simulink model "MotorX_modelling"  (R2020a)
settings: Solver=FixedStepAuto  StartTime=0.0  StopTime=10  RelTol=1e-3  EnableMultiTasking=on
libraries: arduinolib x6, simulink x3, arduinosensorlib x1
settings Model: SILPILModeSetting=veronly  ExtModeTrigDuration=2  Creator=fcemi  LastModifiedBy=fcemi
settings OptimizationCC: EnhancedBackFolding=on  PassReuseOutputArgsAs=Individual arguments  ZeroExternalMemoryAtStartup=off  ZeroInternalMemoryAtStartup=off  MaxStackSize=64  OptimizeBlockOrder=speed  DifferentSizesBufferReuse=on  OptimizationCustomize=off  EfficientTunableParamExpr=on
settings DebuggingCC: ParameterTunabilityLossMsg=error
settings HardwareCC: ProdBitPerInt=16  ProdBitPerPointer=16  ProdBitPerSizeT=16  ProdBitPerPtrDiffT=16  ProdLargestAtomicFloat=None  ProdWordSize=8  ProdHWDeviceType=Atmel->AVR  UseEmbeddedCoderFeatures=off  UseSimulinkCoderFeatures=off
settings SFSimCC: MATLABDynamicMemAlloc=off
settings RTWCC: SystemTargetFile=ert.tlc  HardwareBoard=Arduino Uno  TLCOptions=-aInlineSetEventsForThisBaseRateFcn=TLC_FALSE -aSuppressMultiTaskScheduler=TLC_FALSE -aRateBasedStepFcn=1  TemplateMakefile=ert_default_tmf  Toolchain=Arduino AVR  BuildConfiguration=Faster Runs
settings CodeAppCC: ForceParamTrailComments=on  IgnoreCustomStorageClasses=off  OperatorAnnotations=on  SimulinkDataObjDesc=on  SFDataObjDesc=on  InsertBlockDesc=on
settings ERTTargetCC: SupportContinuousTime=on  SupportNonInlinedSFcns=on  SupportVariableSizeSignals=on  ExtModeStaticAllocSize=250

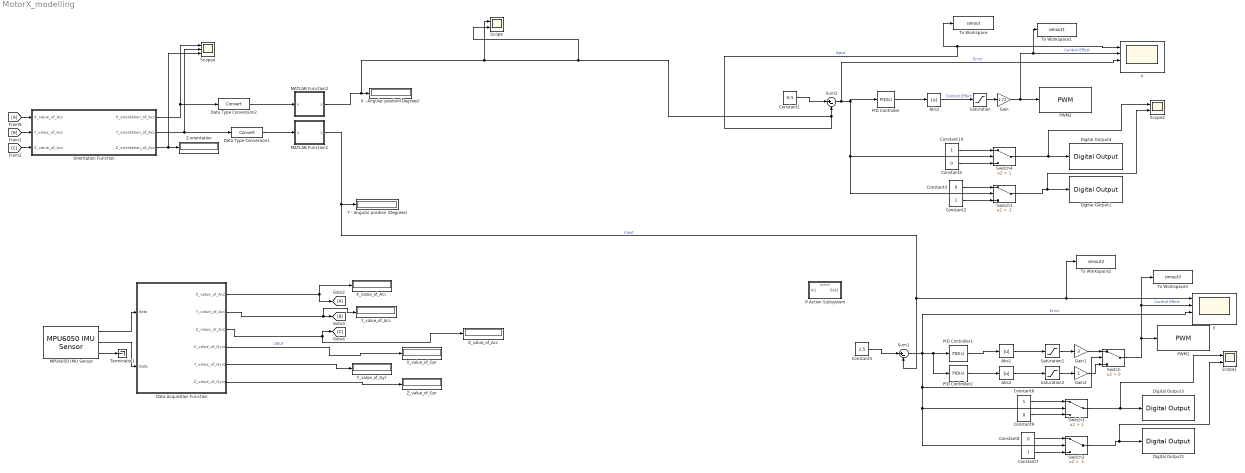
== system MotorX_modelling ==
  Abs1 : Abs
  Abs2 : Abs
  Abs3 : Abs
  Constant1 : Constant  Value=-0.5
  Constant{2,6..7,10} (4 alike) : Constant
  Constant{3..4,8..9} (4 alike) : Constant  Value=0
  Constant5 : Constant  Value=2.5
  Data Acquisition Function : MATLAB Function  TreatAsAtomicUnit=on
  Data Type Conversion1 : DataTypeConversion
  Data Type Conversion2 : DataTypeConversion
  Digital Output1 : arduinolib/Digital Output  pinNumber=8  Direction=output  blockPlatform=arduino
  Digital Output2 : arduinolib/Digital Output  pinNumber=5  Direction=output  blockPlatform=arduino
  Digital Output3 : arduinolib/Digital Output  pinNumber=4  Direction=output  blockPlatform=arduino
  Digital Output4 : arduinolib/Digital Output  pinNumber=9  Direction=output  blockPlatform=arduino
  Gain : Gain  Gain=1.72
  Gain1 : Gain  Gain=3
  Gain2 : Gain
  If Action Subsystem : Subsystem  TreatAsAtomicUnit=on
  MATLAB Function1 : MATLAB Function  TreatAsAtomicUnit=on
  MATLAB Function2 : MATLAB Function  TreatAsAtomicUnit=on
  MPU6050 IMU Sensor : arduinosensorlib/MPU6050 IMU Sensor  SlaveAddress=0x68  Accel=on  AngularRate=on  Temperature=off  Status=on  EulerAngles=off  Quat=off  AccelRange=2G  GyroRange=250 dps  DmpOdr=200 Hz  Dlpf=Accelerometer: 184Hz, Gyroscope: 188Hz  SampleTime=0.01
      settings: SourceProductBaseCode=ARDUINO
  Orientation Function : MATLAB Function  TreatAsAtomicUnit=on
  PID Controller : simulink/Continuous/PID Controller  Controller=PID  Form=Parallel  TimeDomain=Continuous-time  UseExternalTs=off  SampleTime=-1  IntegratorMethod=Forward Euler  FilterMethod=Forward Euler  ControllerParametersSource=internal  P=1  I=0  D=0.01  UseFilter=on  N=100  TunerSelectOption=Transfer Function Based (PID Tuner App)  InitialConditionSource=internal  InitialConditionForIntegrator=0  InitialConditionForFilter=0  DifferentiatorICPrevScaledInput=0  ExternalReset=none  TrackingMode=off  Kt=1  LimitOutput=off  UpperSaturationLimit=inf  LowerSaturationLimit=-inf  LinearizeAsGain=on  AntiWindupMode=none  Kb=1  POutMin=[]  POutMax=[]  IOutMin=[]  IOutMax=[]  DOutMin=[]  DOutMax=[]  NOutMin=[]  NOutMax=[]  SumOutMin=[]  SumOutMax=[]  SaturationOutMin=[]  SaturationOutMax=[]  PParamMin=[]  PParamMax=[]  IParamMin=[]  IParamMax=[]  DParamMin=[]  DParamMax=[]  NParamMin=[]  NParamMax=[]  KbParamMin=[]  KbParamMax=[]  KtParamMin=[]  KtParamMax=[]  KbOutMin=[]  KbOutMax=[]  KtOutMin=[]  KtOutMax=[]  IntegratorOutMin=[]  IntegratorOutMax=[]  FilterOutMin=[]  FilterOutMax=[]  SumI1OutMin=[]  SumI1OutMax=[]  SumI2OutMin=[]  SumI2OutMax=[]  SumI3OutMin=[]  SumI3OutMax=[]  SumI4OutMin=[]  SumI4OutMax=[]  SumDOutMin=[]  SumDOutMax=[]  DifferentiatorOutMin=[]  DifferentiatorOutMax=[]  FilterDiffOutCoefMin=[]  FilterDiffOutCoefMax=[]  ReciprocalOutMin=[]  ReciprocalOutMax=[]  SumDenOutMin=[]  SumDenOutMax=[]  SumNumOutMin=[]  SumNumOutMax=[]  DivideOutMin=[]  DivideOutMax=[]  UdiffTsProdOutMin=[]  UdiffTsProdOutMax=[]  NTsProdOutMin=[]  NTsProdOutMax=[]  UintegralTsProdOutMin=[]  UintegralTsProdOutMax=[]  UngainTsProdOutMin=[]  UngainTsProdOutMax=[]  IntegratorContinuousStateAttributes=''  IntegratorStateMustResolveToSignalObject=off  IntegratorRTWStateStorageClass=Auto  FilterContinuousStateAttributes=''  FilterStateMustResolveToSignalObject=off  FilterRTWStateStorageClass=Auto  ParallelPVariant=InternalParameters  IdealPVariant=Disabled  IVariant=InternalParameters  DVariant=InternalParameters  IntegratorVariant=Continuous  SatVariant=Disabled  AWVariant=Passthrough  PCopyVariant=Disabled  TRVariant=Disabled  FdbkBlocksVariant=Forward  IdealPFdbkVariant=Disabled  SatFdbkVariant=Disabled  DerivativeFilterVariant=ContFilter  NVariant=InternalParameters  NCopyVariant=Disabled  FilterICVariant=InternalICsFilter  IntegratorICVariant=InternalICs  ExternalResetVariant=Disabled  TRSumVariant=Passthrough  SumFdbkVariant=Disabled  SumVariant=Sum_PID  TsampFilterVariant=InternalTs  TsampNgainVariant=Passthrough  TsampIntegralVariant=Passthrough
  PID Controller1 : simulink/Continuous/PID Controller  Controller=PID  Form=Parallel  TimeDomain=Continuous-time  UseExternalTs=off  SampleTime=-1  IntegratorMethod=Forward Euler  FilterMethod=Forward Euler  ControllerParametersSource=internal  P=1  I=0  D=0.01  UseFilter=on  N=100  TunerSelectOption=Transfer Function Based (PID Tuner App)  InitialConditionSource=internal  InitialConditionForIntegrator=0  InitialConditionForFilter=0  DifferentiatorICPrevScaledInput=0  ExternalReset=none  TrackingMode=off  Kt=1  LimitOutput=off  UpperSaturationLimit=inf  LowerSaturationLimit=-inf  LinearizeAsGain=on  AntiWindupMode=none  Kb=1  POutMin=[]  POutMax=[]  IOutMin=[]  IOutMax=[]  DOutMin=[]  DOutMax=[]  NOutMin=[]  NOutMax=[]  SumOutMin=[]  SumOutMax=[]  SaturationOutMin=[]  SaturationOutMax=[]  PParamMin=[]  PParamMax=[]  IParamMin=[]  IParamMax=[]  DParamMin=[]  DParamMax=[]  NParamMin=[]  NParamMax=[]  KbParamMin=[]  KbParamMax=[]  KtParamMin=[]  KtParamMax=[]  KbOutMin=[]  KbOutMax=[]  KtOutMin=[]  KtOutMax=[]  IntegratorOutMin=[]  IntegratorOutMax=[]  FilterOutMin=[]  FilterOutMax=[]  SumI1OutMin=[]  SumI1OutMax=[]  SumI2OutMin=[]  SumI2OutMax=[]  SumI3OutMin=[]  SumI3OutMax=[]  SumI4OutMin=[]  SumI4OutMax=[]  SumDOutMin=[]  SumDOutMax=[]  DifferentiatorOutMin=[]  DifferentiatorOutMax=[]  FilterDiffOutCoefMin=[]  FilterDiffOutCoefMax=[]  ReciprocalOutMin=[]  ReciprocalOutMax=[]  SumDenOutMin=[]  SumDenOutMax=[]  SumNumOutMin=[]  SumNumOutMax=[]  DivideOutMin=[]  DivideOutMax=[]  UdiffTsProdOutMin=[]  UdiffTsProdOutMax=[]  NTsProdOutMin=[]  NTsProdOutMax=[]  UintegralTsProdOutMin=[]  UintegralTsProdOutMax=[]  UngainTsProdOutMin=[]  UngainTsProdOutMax=[]  IntegratorContinuousStateAttributes=''  IntegratorStateMustResolveToSignalObject=off  IntegratorRTWStateStorageClass=Auto  FilterContinuousStateAttributes=''  FilterStateMustResolveToSignalObject=off  FilterRTWStateStorageClass=Auto  ParallelPVariant=InternalParameters  IdealPVariant=Disabled  IVariant=InternalParameters  DVariant=InternalParameters  IntegratorVariant=Continuous  SatVariant=Disabled  AWVariant=Passthrough  PCopyVariant=Disabled  TRVariant=Disabled  FdbkBlocksVariant=Forward  IdealPFdbkVariant=Disabled  SatFdbkVariant=Disabled  DerivativeFilterVariant=ContFilter  NVariant=InternalParameters  NCopyVariant=Disabled  FilterICVariant=InternalICsFilter  IntegratorICVariant=InternalICs  ExternalResetVariant=Disabled  TRSumVariant=Passthrough  SumFdbkVariant=Disabled  SumVariant=Sum_PID  TsampFilterVariant=InternalTs  TsampNgainVariant=Passthrough  TsampIntegralVariant=Passthrough
  PID Controller2 : simulink/Continuous/PID Controller  Controller=PID  Form=Parallel  TimeDomain=Continuous-time  UseExternalTs=off  SampleTime=-1  IntegratorMethod=Forward Euler  FilterMethod=Forward Euler  ControllerParametersSource=internal  P=1  I=0  D=0.01  UseFilter=on  N=100  TunerSelectOption=Transfer Function Based (PID Tuner App)  InitialConditionSource=internal  InitialConditionForIntegrator=0  InitialConditionForFilter=0  DifferentiatorICPrevScaledInput=0  ExternalReset=none  TrackingMode=off  Kt=1  LimitOutput=off  UpperSaturationLimit=inf  LowerSaturationLimit=-inf  LinearizeAsGain=on  AntiWindupMode=none  Kb=1  POutMin=[]  POutMax=[]  IOutMin=[]  IOutMax=[]  DOutMin=[]  DOutMax=[]  NOutMin=[]  NOutMax=[]  SumOutMin=[]  SumOutMax=[]  SaturationOutMin=[]  SaturationOutMax=[]  PParamMin=[]  PParamMax=[]  IParamMin=[]  IParamMax=[]  DParamMin=[]  DParamMax=[]  NParamMin=[]  NParamMax=[]  KbParamMin=[]  KbParamMax=[]  KtParamMin=[]  KtParamMax=[]  KbOutMin=[]  KbOutMax=[]  KtOutMin=[]  KtOutMax=[]  IntegratorOutMin=[]  IntegratorOutMax=[]  FilterOutMin=[]  FilterOutMax=[]  SumI1OutMin=[]  SumI1OutMax=[]  SumI2OutMin=[]  SumI2OutMax=[]  SumI3OutMin=[]  SumI3OutMax=[]  SumI4OutMin=[]  SumI4OutMax=[]  SumDOutMin=[]  SumDOutMax=[]  DifferentiatorOutMin=[]  DifferentiatorOutMax=[]  FilterDiffOutCoefMin=[]  FilterDiffOutCoefMax=[]  ReciprocalOutMin=[]  ReciprocalOutMax=[]  SumDenOutMin=[]  SumDenOutMax=[]  SumNumOutMin=[]  SumNumOutMax=[]  DivideOutMin=[]  DivideOutMax=[]  UdiffTsProdOutMin=[]  UdiffTsProdOutMax=[]  NTsProdOutMin=[]  NTsProdOutMax=[]  UintegralTsProdOutMin=[]  UintegralTsProdOutMax=[]  UngainTsProdOutMin=[]  UngainTsProdOutMax=[]  IntegratorContinuousStateAttributes=''  IntegratorStateMustResolveToSignalObject=off  IntegratorRTWStateStorageClass=Auto  FilterContinuousStateAttributes=''  FilterStateMustResolveToSignalObject=off  FilterRTWStateStorageClass=Auto  ParallelPVariant=InternalParameters  IdealPVariant=Disabled  IVariant=InternalParameters  DVariant=InternalParameters  IntegratorVariant=Continuous  SatVariant=Disabled  AWVariant=Passthrough  PCopyVariant=Disabled  TRVariant=Disabled  FdbkBlocksVariant=Forward  IdealPFdbkVariant=Disabled  SatFdbkVariant=Disabled  DerivativeFilterVariant=ContFilter  NVariant=InternalParameters  NCopyVariant=Disabled  FilterICVariant=InternalICsFilter  IntegratorICVariant=InternalICs  ExternalResetVariant=Disabled  TRSumVariant=Passthrough  SumFdbkVariant=Disabled  SumVariant=Sum_PID  TsampFilterVariant=InternalTs  TsampNgainVariant=Passthrough  TsampIntegralVariant=Passthrough
  PWM1 : arduinolib/PWM  pinNumber=3  frequencyType=Default  desiredFrequency=490.2  achievableFrequency=490.2
  PWM2 : arduinolib/PWM  pinNumber=10  frequencyType=Default  desiredFrequency=490.2  achievableFrequency=490.2
  Saturation : Saturate  UpperLimit=28  LowerLimit=18
  Saturation1 : Saturate  UpperLimit=27  LowerLimit=20
  Saturation2 : Saturate  UpperLimit=20  LowerLimit=0
  Scope : Scope  NumInputPorts=2
  Scope1 : Scope  NumInputPorts=2
  Scope2 : Scope  NumInputPorts=2
  Scope4 : Scope  NumInputPorts=3
  Sum1 : Sum  Inputs=|+-
  Sum2 : Sum  Inputs=|+-
  Switch : Switch  Criteria=u2 > Threshold
  Switch1 : Switch  Criteria=u2 > Threshold  Threshold=-1
  Switch2 : Switch  Criteria=u2 > Threshold  Threshold=-1
  Switch3 : Switch  Criteria=u2 > Threshold  Threshold=1
  Switch4 : Switch  Criteria=u2 > Threshold  Threshold=1
  Terminator1 : Terminator
  To Workspace : ToWorkspace  VariableName=simout  SaveFormat=Timeseries  SampleTime=-1
  To Workspace1 : ToWorkspace  VariableName=simout1  SaveFormat=Timeseries  SampleTime=-1
  To Workspace2 : ToWorkspace  VariableName=simout2  SaveFormat=Timeseries  SampleTime=-1
  To Workspace3 : ToWorkspace  VariableName=simout3  SaveFormat=Timeseries  SampleTime=-1
  X - Angular position(Degrees) : Display
  X_value_of_Acc : Display
      settings: Format=bank
  X_value_of_Gyr : Display
      settings: Format=bank
  Y - Angular position (Degrees) : Display
  Y_value_of_Acc : Display
      settings: Format=bank
  Y_value_of_Gyr : Display
      settings: Format=bank
  Z-orientation : Display
      settings: Format=bank
  Z_value_of_Acc : Display
      settings: Format=bank
  Z_value_of_Gyr : Display
      settings: Format=bank
  x : Scope  NumInputPorts=4
  y : Scope  NumInputPorts=4
  wires:
  Orientation Function/3(Z_orientation_of_Acc) -> Scope4/3, Z-orientation/1
  [A] -> Orientation Function/1(X_value_of_Acc)
  [C] -> Orientation Function/3(Z_value_of_Acc)
  Orientation Function/2(Y_orientation_of_Acc) -> Data Type Conversion1/1, Scope4/2
  [B] -> Orientation Function/2(Y_value_of_Acc)
  Data Type Conversion2/1 -> MATLAB Function2/1(u)
  Data Type Conversion1/1 -> MATLAB Function1/1(u)
  Orientation Function/1(X_orientation_of_Acc) -> Scope4/1, Data Type Conversion2/1
  Constant2/1 -> Switch1/3
  Constant10/1 -> Switch4/1
  Switch4/1 -> Scope2/1, Digital Output4/1
  Abs2/1 -> Saturation/1  "Control Effort"
  Constant3/1 -> Switch1/1
  Switch1/1 -> Scope2/2, Digital Output1/1
  Constant4/1 -> Switch4/3
  Sum2/1 -> x/3, PID Controller/1, Switch1/2, Switch4/2  "Error"
  MATLAB Function2/1(y) -> Scope/2, Sum2/2, x/1, To Workspace/1, Scope/1, X - Angular position(Degrees)/1  "Input"
  Constant1/1 -> Sum2/1
  Data Acquisition Function/5(Y_value_of_Gyro) -> Y_value_of_Gyr/1
  MPU6050 IMU Sensor/3 -> Terminator1/1
  Data Acquisition Function/1(X_value_of_Acc) -> [A], X_value_of_Acc/1
  MPU6050 IMU Sensor/1 -> Data Acquisition Function/1(data)
  Data Acquisition Function/6(Z_value_of_Gyro) -> Z_value_of_Gyr/1
  Data Acquisition Function/4(X_value_of_Gyro) -> X_value_of_Gyr/1  "utput"
  MPU6050 IMU Sensor/2 -> Data Acquisition Function/2(Data)
  Data Acquisition Function/2(Y_value_of_Acc) -> Y_value_of_Acc/1, [B]
  Data Acquisition Function/3(Z_value_of_Acc) -> Z_value_of_Acc/1, [C]
  Constant5/1 -> Sum1/1
  Constant8/1 -> Switch2/1
  Switch3/1 -> Scope1/1, Digital Output3/1
  Sum1/1 -> y/3, PID Controller2/1, PID Controller1/1, Switch/2, Switch2/2, Switch3/2  "Error"
  MATLAB Function1/1(y) -> Sum1/2, y/1, To Workspace2/1, Y - Angular position (Degrees)/1  "Input"
  Switch2/1 -> Scope1/2, Digital Output2/1
  Constant9/1 -> Switch3/3
  Constant6/1 -> Switch3/1
  Abs1/1 -> Saturation1/1
  Constant7/1 -> Switch2/3
  PID Controller1/1 -> Abs1/1
  Saturation/1 -> Gain/1
  Gain/1 -> PWM2/1, To Workspace1/1, x/2  "Control Effort"
  PID Controller/1 -> Abs2/1
  Saturation1/1 -> Gain1/1
  Saturation2/1 -> Gain2/1
  Gain1/1 -> Switch/1
  Gain2/1 -> Switch/3
  Switch/1 -> To Workspace3/1, y/2, PWM1/1  "Control Effort"
  Abs3/1 -> Saturation2/1
  PID Controller2/1 -> Abs3/1

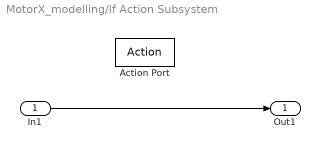
== system MotorX_modelling/If Action Subsystem ==
  In1 : Inport
  Action Port : ActionPort
  Out1 : Outport
  wires:
  In1/1 -> Out1/1

== matlab function MotorX_modelling/Data Acquisition Function ==
  data: data input; Data input; X_value_of_Acc output; Y_value_of_Acc output; Z_value_of_Acc output; X_value_of_Gyro output; Y_value_of_Gyro output; Z_value_of_Gyro output
% Reading IMU packet bytes from Sensor Stream App 
% Author: RM van Rensburg
% Date: 26-04-2015
% Version: 1.0,tested on Matlab R2015a

function [X_value_of_Acc,Y_value_of_Acc, Z_value_of_Acc,...
          X_value_of_Gyro, Y_value_of_Gyro, Z_value_of_Gyro]...
          = fcn(data, Data)
             
% Header packet
% Header = Data(1:4);

% Accelerometer data
X_value_of_Acc = data(1,:);
Y_value_of_Acc = data(2,:);
Z_value_of_Acc = data(3,:);

% Gyroscope data
X_value_of_Gyro = Data(1,:);
Y_value_of_Gyro = Data(2,:);
Z_value_of_Gyro = Data(3,:);

% Proximity sensor
% X_value_of_Tes = typecast(uint8(Data(29:36)),'double');
% Y_value_of_Tes = typecast(uint8(Data(37:44)),'double');
% Z_value_of_Tes = typecast(uint8(Data(45:52)),'double');

== matlab function MotorX_modelling/MATLAB Function2 ==
  data: u input; y output
function y = fcn(u)

if(isnan(u))
y=0;
else
y=u;
end

== matlab function MotorX_modelling/Orientation Function ==
  data: X_value_of_Acc input; X_orientation_of_Acc output; Y_orientation_of_Acc output; Z_orientation_of_Acc output; Y_value_of_Acc input; Z_value_of_Acc input
% Computing orientation of tri-axial acclerometer data from IMU 
% Author: RM van Rensburg
% Date: 26-04-2015
% Version: 1.0,tested on Matlab R2015a

function [X_orientation_of_Acc,...
          Y_orientation_of_Acc,...
          Z_orientation_of_Acc]...
          = OrientationFcn(X_value_of_Acc,Y_value_of_Acc,Z_value_of_Acc)
     
      
% Using x and y from accelerometer (g-forces), calculate x and y angles
% Data directly obtained from IMU
% Using the following formulae
% Ax = arctan{X/sqrt(Y*Y + Z*Z)}
% Ay = arctan{Y/sqrt(X*X + Z*Z)}

% Computing the X*X, Y*Y, Z*Z
X2 = power(X_value_of_Acc,2);
Y2 = power(Y_value_of_Acc,2);
Z2 = power(Z_value_of_Acc,2);

% x-axis angle
result = sqrt(Y2 + Z2);
result = X_value_of_Acc / result;
x_angle_rad = atan(result);
X_orientation_of_Acc = (x_angle_rad * 180) / pi;

% y-axis angle
result = sqrt(X2 + Z2);
result = Y_value_of_Acc / result;
y_angle_rad = atan(result);
Y_orientation_of_Acc = (y_angle_rad * 180) / pi;

% z-axis angle
result = sqrt(Y2 + X2);
result = Z_value_of_Acc / result;
z_angle_rad = atan(result);
Z_orientation_of_Acc = (z_angle_rad * 180) / pi;

end

== matlab function MotorX_modelling/MATLAB Function1 ==
  data: u input; y output
function y = fcn(u)

if(isnan(u))
y=0;
else
y=u;
end
